simulink model "SistemaLineal1"  (R2018b)
settings: Solver=VariableStepAuto  StartTime=0.0  StopTime=ttotal  RelTol=1e-3
values from neighbouring files (symbols this model uses):
  iseed = randi(2^53-1)    [IdentificacionTS.m]
  tmuestra = 0.2    [ControlDeEstadosTS.m]    (also in IdentificacionTS.m = 0.02; MultiTestTS.m = 0.02)
  var = 0.001    [IdentificacionTS.m]
undefined symbols (not defined in the file or in its folder): denom1, denom2, num1, num2
settings Model: Creator=pablo  LastModifiedBy=pablo

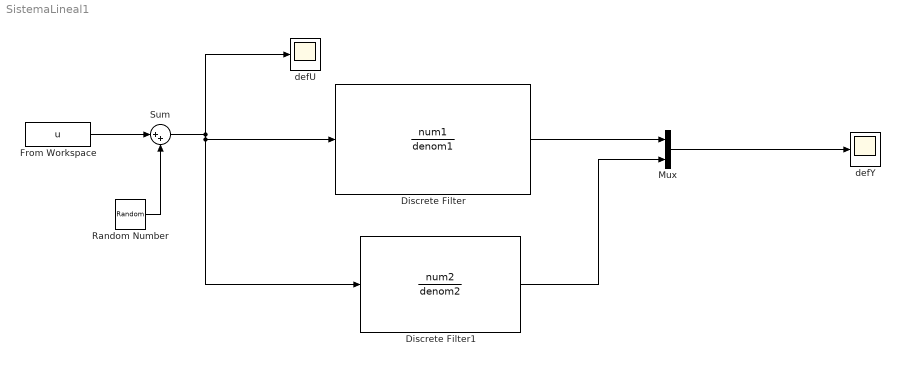
== system SistemaLineal1 ==
  Discrete Filter : DiscreteFilter  Numerator=num1  Denominator=denom1
  Discrete Filter1 : DiscreteFilter  Numerator=num2  Denominator=denom2
  From Workspace : FromWorkspace  VariableName=u  SampleTime=tmuestra
  Mux : Mux  Inputs=2
  Random Number : RandomNumber  Variance=var  Seed=iseed  SampleTime=tmuestra
  Sum : Sum  Inputs=|++
  "defU " : Scope
  "defY " : Scope
  wires:
  From Workspace/1 -> Sum/1
  Random Number/1 -> Sum/2
  Sum/1 -> Discrete Filter1/1, Discrete Filter/1, "defU "/1
  Discrete Filter/1 -> Mux/1
  Discrete Filter1/1 -> Mux/2
  Mux/1 -> "defY "/1
